simulink model "SerialSendReceive_etiqueta"  (R2020b)
settings: Solver=FixedStepDiscrete  StartTime=0.0  StopTime=inf  FixedStep=0.01  RelTol=1e-3
libraries: arduinolib x4, commutil2 x1
settings Model: SimulationMode=external  ExtModeTrigDuration=2  Creator=Pablo  LastModifiedBy=manol
settings SolverCC: AutoInsertRateTranBlk=on
settings DataIOCC: ReturnWorkspaceOutputs=off
settings OptimizationCC: PassReuseOutputArgsAs=Individual arguments  MaxStackSize=64  EfficientTunableParamExpr=on
settings DebuggingCC: ParameterOverflowMsg=none  ParameterTunabilityLossMsg=error  ArithmeticOperatorsInVariantConditions=warning
settings HardwareCC: ProdBitPerInt=16  ProdBitPerPointer=16  ProdBitPerSizeT=16  ProdBitPerPtrDiffT=16  ProdLargestAtomicFloat=None  ProdWordSize=8  ProdHWDeviceType=Atmel->AVR  UseEmbeddedCoderFeatures=off  UseSimulinkCoderFeatures=off
settings SFSimCC: SimUseLocalCustomCode=off  MATLABDynamicMemAlloc=off  CustomCodeUndefinedFunction=UseInterfaceOnly
settings RTWCC: Description=Embedded Coder  SystemTargetFile=ert.tlc  HardwareBoard=Arduino Mega 2560  TemplateMakefile=ert_default_tmf  RTWVerbose=off  RTWUseLocalCustomCode=off  Toolchain=Arduino AVR  BuildConfiguration=Faster Runs  IncludeHyperlinkInReport=on
settings CodeAppCC: ForceParamTrailComments=on  OperatorAnnotations=on  SimulinkDataObjDesc=on  SFDataObjDesc=on  MangleLength=10  InsertBlockDesc=on
settings ERTTargetCC: SupportContinuousTime=on  SupportNonInlinedSFcns=on  SupportVariableSizeSignals=on  ExtMode=on  ExtModeMexArgs='127.0.0.1' 0 17725  ERTSrcFileBannerTemplate=codertarget_code_template.cgt  ERTHdrFileBannerTemplate=codertarget_code_template.cgt  ERTDataSrcFileTemplate=codertarget_code_template.cgt  ERTDataHdrFileTemplate=codertarget_code_template.cgt

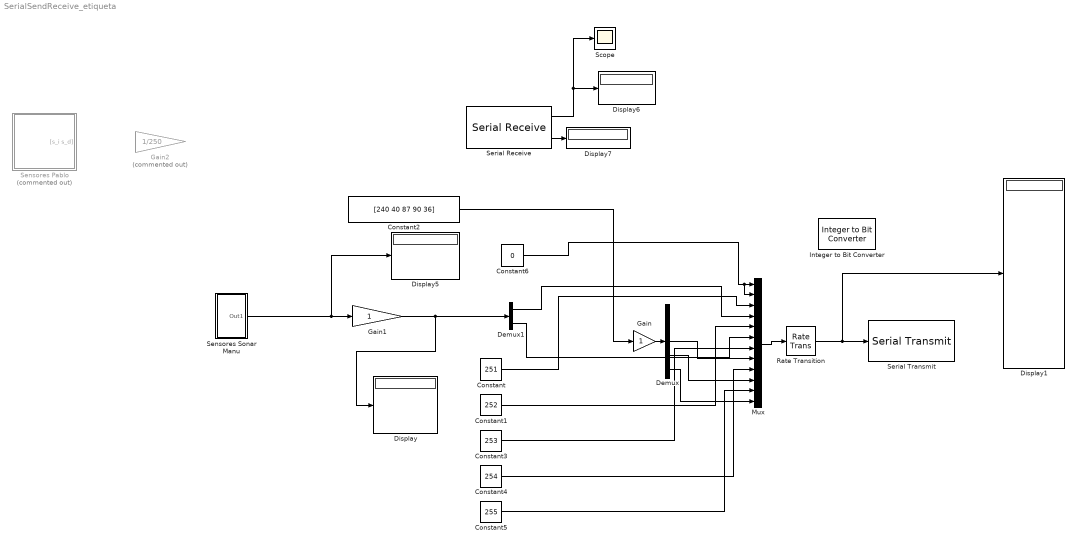
== system SerialSendReceive_etiqueta ==
  Constant : Constant  Value=251  OutDataTypeStr=uint8
  Constant1 : Constant  Value=252  OutDataTypeStr=uint8
  Constant2 : Constant  Value=[240 40 87 90 36]  OutDataTypeStr=double
  Constant3 : Constant  Value=253  OutDataTypeStr=uint8
  Constant4 : Constant  Value=254  OutDataTypeStr=uint8
  Constant5 : Constant  Value=255  OutDataTypeStr=uint8
  Constant6 : Constant  Value=0  OutDataTypeStr=uint8
  Demux : Demux  Outputs=5
  Demux1 : Demux  Outputs=2
  Display{,1,5..7} (5 alike) : Display
  Gain : Gain  OutMax=250  OutDataTypeStr=uint8
  Gain1 : Gain  OutDataTypeStr=uint8
  Gain2 : Gain  Commented=on  Gain=1/250  OutDataTypeStr=uint8
  Integer to Bit Converter : commutil2/Integer to Bit Converter  nbits=3  signedInputValues=Unsigned  bitOrder=MSB first  outDtype=Inherit via internal rule
  Mux : Mux  Inputs=12
  Rate Transition : RateTransition  OutPortSampleTime=1
  Scope : Scope
  Sensores Pablo : Subsystem  Commented=on
      mask Display: image('C:\Users\Lenovo\Desktop\4ºGIERM\LAB ROB\sensor.jpg'); % Use "Edit Image" on toolstrip to change.
  Sensores Sonar Manu : Subsystem
  Serial Receive : arduinolib/Serial Receive  isARMArch=off  portNumber=3  DataType=uint8  Datalength=2  SampleTime=0.1  showOutStatus=on  blockPlatform=arduino
      settings: SourceProductBaseCode=ARDUINO
  Serial Transmit : arduinolib/Serial Transmit  portNumber=3  sendmode=write  label=sensores  sendformat=Decimal  floatprecision=2  blockPlatform=arduino
  wires:
  Serial Receive/1 -> Scope/1, Display6/1
  Serial Receive/2 -> Display7/1
  Constant2/1 -> Gain/1
  Rate Transition/1 -> Display1/1, Serial Transmit/1
  Gain/1 -> Demux/1
  Demux/3 -> Mux/8
  Demux/4 -> Mux/10
  Demux/5 -> Mux/12
  Constant/1 -> Mux/3
  Constant1/1 -> Mux/5
  Constant3/1 -> Mux/7
  Constant4/1 -> Mux/9
  Constant5/1 -> Mux/11
  Mux/1 -> Rate Transition/1
  Constant6/1 -> Mux/2, Mux/1
  Demux1/1 -> Mux/4
  Demux1/2 -> Mux/6
  Gain1/1 -> Display/1, Demux1/1
  Sensores Sonar Manu/1(Out1) -> Display5/1, Gain1/1

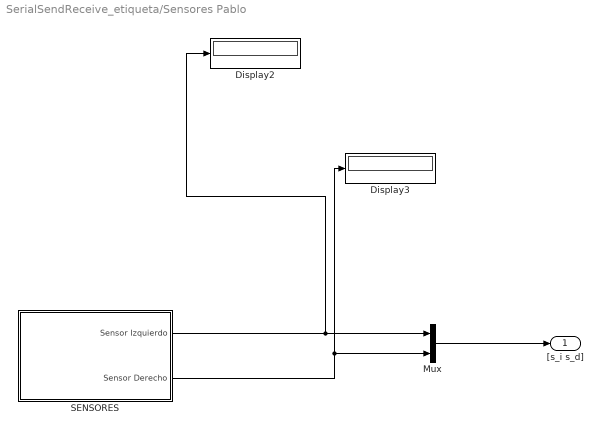
== system SerialSendReceive_etiqueta/Sensores Pablo ==
  Display2 : Display
  Display3 : Display
  Mux : Mux  Inputs=2
  SENSORES : Subsystem
  "[s_i s_d]" : Outport
  wires:
  SENSORES/2(Sensor Derecho) -> Mux/2, Display3/1
  SENSORES/1(Sensor Izquierdo) -> Mux/1, Display2/1
  Mux/1 -> "[s_i s_d]"/1

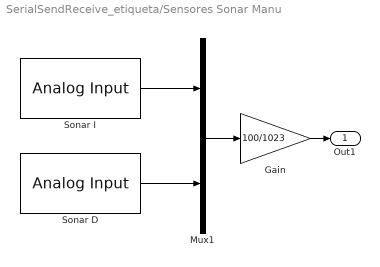
== system SerialSendReceive_etiqueta/Sensores Sonar Manu ==
  Gain : Gain  Gain=100/1023
  Mux1 : Mux  Inputs=2
  Sonar D : arduinolib/Analog Input  pinNumber=0  ReadResultsOnly=off  ConversionTriggerSource=Software  ExternalTriggerType=uint32( 0 )  OutputDataType=uint16  EnableConversionCompleteNotify=off  EnableOuputStatus=off  SampleTime=0.1  blockPlatform=arduino
  Sonar I : arduinolib/Analog Input  pinNumber=1  ReadResultsOnly=off  ConversionTriggerSource=Software  ExternalTriggerType=uint32( 0 )  OutputDataType=uint16  EnableConversionCompleteNotify=off  EnableOuputStatus=off  SampleTime=0.1  blockPlatform=arduino
  Out1 : Outport  VectorParamsAs1DForOutWhenUnconnected=off
  wires:
  Gain/1 -> Out1/1
  Mux1/1 -> Gain/1
  Sonar I/1 -> Mux1/1
  Sonar D/1 -> Mux1/2

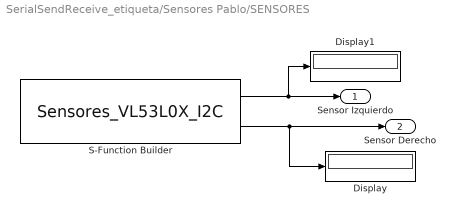
== system SerialSendReceive_etiqueta/Sensores Pablo/SENSORES ==
  Display : Display
  Display1 : Display
  S-Function Builder : S-Function  InitFcn=try, set_param(gcb,'FunctionName','Sensores_VL53L0X_I2C'), end  FunctionName=Sensores_VL53L0X_I2C  SFunctionModules=Sensores_VL53L0X_I2C_wrapper  SFunctionDeploymentMode=off  EnableBusSupport=off  mask(S-Function Builder){}
      mask help: Simulink:masks:SFunctionBuilder_MD
      mask init:
      | val = [[.9  0.75 0.75 1 1 .9 .9 1]',[1 1 0.75 0.75 .9 .9 1 .9]'];try , sys = get_param(gcb,'SfunBuilderFcnName');if isempty(sys), sys = get_param(gcb,'FunctionName'); end,catch, sys = get_param(gcb,'FunctionName'); end
      settings: CopyFcn=set_param(gcbh,'LinkStatus','none')  PreSaveFcn=try, set_param(gcb,'FunctionName','Sensores_VL53L0X_I2C'), end  OpenFcn=sfunctionwizard(gcbh)
      mask Display:
      | plot(val(:,1),val(:,2))
      | disp(sys)
      | port_label('output',1,'Sensor1')
      | port_label('output',2,'Sensor2')
  Sensor Izquierdo : Outport  VectorParamsAs1DForOutWhenUnconnected=off
  Sensor Derecho : Outport  Port=2  VectorParamsAs1DForOutWhenUnconnected=off
  wires:
  S-Function Builder/2 -> Display/1, Sensor Derecho/1
  S-Function Builder/1 -> Display1/1, Sensor Izquierdo/1
